simulink model "sim_orb_ctrl_1"  (R2022a)
settings: Solver=ode4  StartTime=0.0  StopTime=Tfin  FixedStep=st_size  RelTol=1e-3
values from neighbouring files (symbols this model uses):
  K = nmpc_design_st(par)    [main_launch.m]
  st_size = 1    [main_launch.m]
  x0 = [RE 0 0 0 0.465 0 m0]'    [main_launch.m]
  yr = [ar;er;cir]    [main_launch.m]
undefined symbols (not defined in the file or in its folder): orbit_animation, rv2oe, spacecraft_dynamics
settings Model: Creator=carlonovara  LastModifiedBy=carlonovara
settings SolverCC: AlgebraicLoopSolver=TrustRegion
settings DataIOCC: ReturnWorkspaceOutputs=off
settings DebuggingCC: UnconnectedInputMsg=warning  UnconnectedOutputMsg=warning  UnconnectedLineMsg=warning  SFMachineParentedDataDiag=warning  ArithmeticOperatorsInVariantConditions=warning
settings SFSimCC: SimUseLocalCustomCode=off  CustomCodeUndefinedFunction=UseInterfaceOnly
settings RTWCC: RTWUseLocalCustomCode=off  DLArmComputeVersion=19.05
settings CodeAppCC: StateflowObjectComments=on

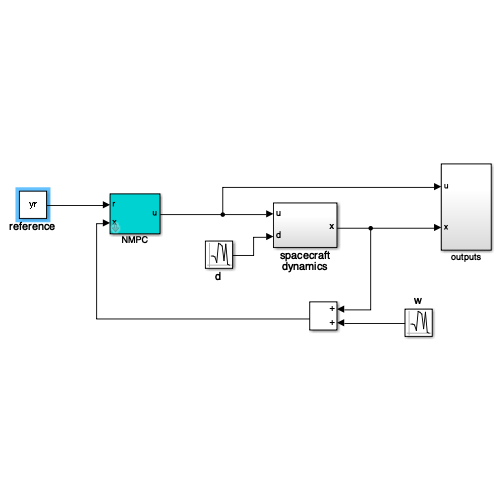
[thumbnail: Simulink's stored preview of the top-level diagram]
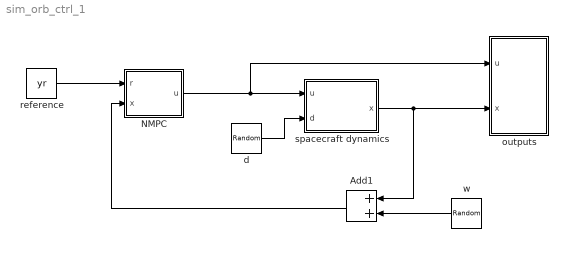
== system sim_orb_ctrl_1 ==
  Add1 : Sum
  NMPC : Subsystem  mask{K=K}
      mask prompts: K "NMPC structure"
  d : RandomNumber  Mean=zeros(3,1)  Variance=1e-4*ones(3,1)  Seed=3689  SampleTime=st_size
  outputs : Subsystem
  reference : Constant  Value=yr
  spacecraft dynamics : Subsystem
  w : RandomNumber  Mean=zeros(7,1)  Variance=[1e-6*ones(3,1);1e-8*ones(3,1);1e-6]  Seed=765  SampleTime=st_size
  wires:
  reference/1 -> NMPC/1(r)
  Add1/1 -> NMPC/2(x)
  w/1 -> Add1/2
  NMPC/1(u) -> outputs/1(u), spacecraft dynamics/1(u)
  d/1 -> spacecraft dynamics/2(d)
  spacecraft dynamics/1(x) -> Add1/1, outputs/2(x)

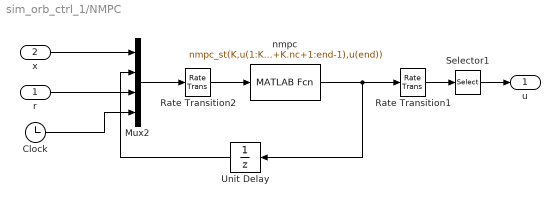
== system sim_orb_ctrl_1/NMPC ==
  r : Inport
  x : Inport  Port=2
  Clock : Clock
  Mux2 : Mux
  Rate Transition1 : RateTransition  OutPortSampleTime=K.Ts
  Rate Transition2 : RateTransition  OutPortSampleTime=K.Ts
  Selector1 : Selector  InputPortWidth=K.nc  IndexOptions=Index vector (dialog)  Indices=1:K.nu  OutputSizes=1
  Unit Delay : UnitDelay  InitialCondition=zeros(K.nc,1)  SampleTime=K.Ts  HasFrameUpgradeWarning=on
  nmpc : MATLABFcn  MATLABFcn=nmpc_st(K,u(1:K.nx),u(K.nx+1:K.nx+K.nc),u(K.nx+K.nc+1:end-1),u(end))  OutputDimensions=K.nc
  u : Outport
  wires:
  Selector1/1 -> u/1
  Unit Delay/1 -> Mux2/2
  nmpc/1 -> Unit Delay/1, Rate Transition1/1
  Rate Transition1/1 -> Selector1/1
  Mux2/1 -> Rate Transition2/1
  x/1 -> Mux2/1
  r/1 -> Mux2/3
  Clock/1 -> Mux2/4
  Rate Transition2/1 -> nmpc/1

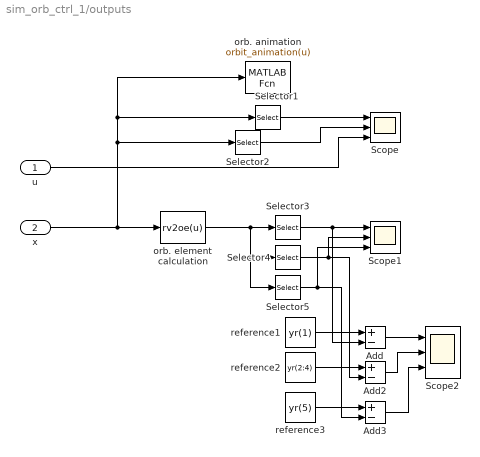
== system sim_orb_ctrl_1/outputs ==
  u : Inport
  x : Inport  Port=2
  Add : Sum  Inputs=+-
  Add2 : Sum  Inputs=+-
  Add3 : Sum  Inputs=+-
  Scope : Scope  NumInputPorts=3
  Scope1 : Scope  NumInputPorts=3
  Scope2 : Scope  NumInputPorts=3
  Selector1 : Selector  InputPortWidth=7  IndexOptions=Index vector (dialog)  Indices=1:3  OutputSizes=1
  Selector2 : Selector  InputPortWidth=7  IndexOptions=Index vector (dialog)  Indices=7  OutputSizes=1
  Selector3 : Selector  InputPortWidth=5  IndexOptions=Index vector (dialog)  Indices=1  OutputSizes=1
  Selector4 : Selector  InputPortWidth=5  IndexOptions=Index vector (dialog)  Indices=2:4  OutputSizes=1
  Selector5 : Selector  InputPortWidth=5  IndexOptions=Index vector (dialog)  Indices=5  OutputSizes=1
  orb. animation : MATLABFcn  MATLABFcn=orbit_animation(u)  OutputDimensions=0
  orb. element calculation : MATLABFcn  MATLABFcn=rv2oe(u)  OutputDimensions=5
  reference1 : Constant  Value=yr(1)
  reference2 : Constant  Value=yr(2:4)
  reference3 : Constant  Value=yr(5)
  wires:
  u/1 -> Scope/3
  Add3/1 -> Scope2/3
  Selector2/1 -> Scope/2
  Selector4/1 -> Add2/2, Scope1/2
  Selector1/1 -> Scope/1
  reference1/1 -> Add/1
  reference2/1 -> Add2/1
  Add2/1 -> Scope2/2
  Selector3/1 -> Add/2, Scope1/1
  reference3/1 -> Add3/1
  orb. element calculation/1 -> Selector5/1, Selector4/1, Selector3/1
  Selector5/1 -> Add3/2, Scope1/3
  Add/1 -> Scope2/1
  x/1 -> Selector2/1, orb. animation/1, Selector1/1, orb. element calculation/1

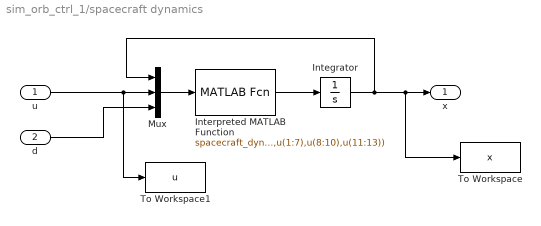
== system sim_orb_ctrl_1/spacecraft dynamics ==
  u : Inport
  d : Inport  Port=2
  Integrator : Integrator  InitialCondition=x0
  Interpreted MATLAB Function : MATLABFcn  MATLABFcn=spacecraft_dynamics(0,u(1:7),u(8:10),u(11:13))
  Mux : Mux  Inputs=3
  To Workspace : ToWorkspace  VariableName=x  SaveFormat=Timeseries  SampleTime=-1
  To Workspace1 : ToWorkspace  VariableName=u  SaveFormat=Timeseries  SampleTime=-1
  x : Outport  VectorParamsAs1DForOutWhenUnconnected=off
  wires:
  Mux/1 -> Interpreted MATLAB Function/1
  Integrator/1 -> Mux/1, To Workspace/1, x/1
  Interpreted MATLAB Function/1 -> Integrator/1
  u/1 -> To Workspace1/1, Mux/2
  d/1 -> Mux/3
